simulink model "sl_subsys_sw1"  (Simulink 6.0)
settings: Solver=FixedStepDiscrete  SolverMode=SingleTasking  StartTime=0.0  StopTime=500  FixedStep=0.001  RelTol=1e-3
settings Model: CovMetricSettings=d  Creator=The MathWorks Inc.  LastModifiedBy=batserve  ExtModeAutoUpdateStatusClock=off
settings DataIOCC: SignalLoggingName=sigsOut
settings OptimizationCC: BlockReduction=off  BooleanDataType=off
settings DebuggingCC: CheckExecutionContextPreStartOutputMsg=on  CheckExecutionContextRuntimeOutputMsg=on  SolverPrmCheckMsg=none
settings HardwareCC: TargetUnknown=on

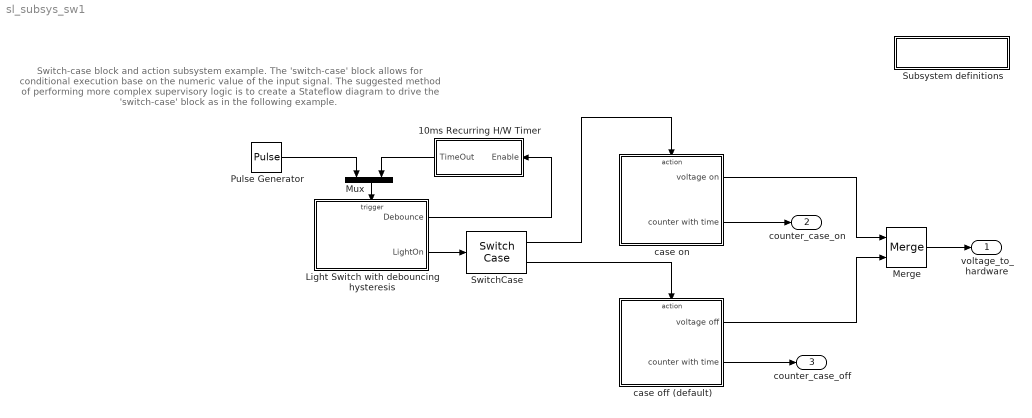
== system sl_subsys_sw1 ==
  note: Switch-case block and action subsystem example.
      |
      | The 'switch-case' block allows for conditional execution base on the numeric value
      | of the input signal. The suggested method of performing more complex supervisory
      | logic is to create a Stateflow diagram to drive the 'switch-case' block as in the
      | following example.
  " Subsystem definitions" : Subsystem  PropExecContextAcrossSSBoundary=on
      settings: OpenFcn=helpview([matlabroot,'/toolbox/simulink/simdemos/sl_subsys_definitions.html']);
      mask Display: disp('Subsystem\ndefinitions')
  10ms Recurring H/W Timer : Subsystem  Orientation=left  PropExecContextAcrossSSBoundary=on
  Light Switch with debouncing hysteresis : Stateflow chart  TreatAsAtomicUnit=on  PropExecContextAcrossSSBoundary=on
  Merge : Merge
  Mux : Mux  Orientation=down  Inputs=2
  Pulse Generator : DiscretePulseGenerator  Period=[64]  PulseWidth=[1]  PhaseDelay=1
  SwitchCase : SwitchCase
  case off (default) : Subsystem  TreatAsAtomicUnit=on  PropExecContextAcrossSSBoundary=on
  case on : Subsystem  TreatAsAtomicUnit=on  PropExecContextAcrossSSBoundary=on
  voltage_to_hardware : Outport
  counter_case_on : Outport  Port=2
  counter_case_off : Outport  Port=3
  wires:
  SwitchCase/1 -> case on/Action
  case on/1(voltage on) -> Merge/1
  case off (default)/1(voltage off) -> Merge/2
  Merge/1 -> voltage_to_hardware/1
  case on/2(counter with time) -> counter_case_on/1
  case off (default)/2(counter with time) -> counter_case_off/1
  Light Switch with debouncing hysteresis/2(LightOn) -> SwitchCase/1
  Light Switch with debouncing hysteresis/1(Debounce) -> 10ms Recurring H/W Timer/1(Enable)
  Mux/1 -> Light Switch with debouncing hysteresis/Trigger
  Pulse Generator/1 -> Mux/1
  10ms Recurring H/W Timer/1(TimeOut) -> Mux/2
  SwitchCase/2 -> case off (default)/Action

== system sl_subsys_sw1/ Subsystem definitions ==

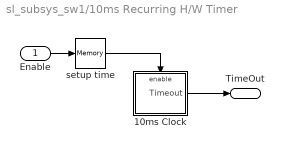
== system sl_subsys_sw1/10ms Recurring H/W Timer ==
  Enable : Inport  Port=1  LatchInput=off
  10ms Clock : Subsystem  TreatAsAtomicUnit=on  PropExecContextAcrossSSBoundary=on
  setup time : Memory  InheritSampleTime=on
  TimeOut : Outport
  wires:
  Enable/1 -> setup time/1
  10ms Clock/1(Timeout) -> TimeOut/1
  setup time/1 -> 10ms Clock/Enable

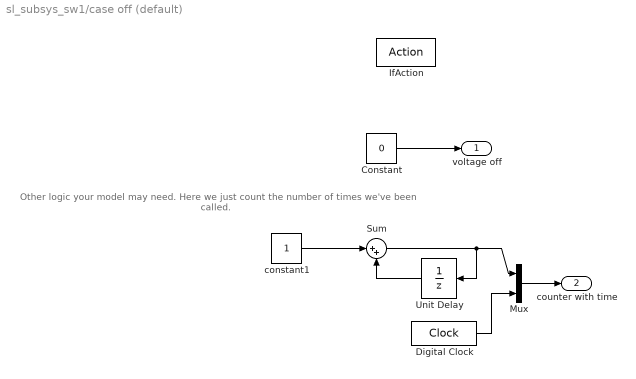
== system sl_subsys_sw1/case off (default) ==
  note: Other logic your model may need. Here we just count the number
      | of times we've been called.
  IfAction : ActionPort  ActionType=default
  Constant : Constant  Value=0
  Digital Clock : DigitalClock
  Mux : Mux  Inputs=2
  Sum : Sum  Inputs=|++  SaturateOnIntegerOverflow=on  InputSameDT=on
  Unit Delay : UnitDelay  Orientation=left
  constant1 : Constant
  voltage off : Outport
  counter with time : Outport  Port=2
  wires:
  Digital Clock/1 -> Mux/2
  Mux/1 -> counter with time/1
  Unit Delay/1 -> Sum/2
  constant1/1 -> Sum/1
  Sum/1 -> Unit Delay/1, Mux/1
  Constant/1 -> voltage off/1

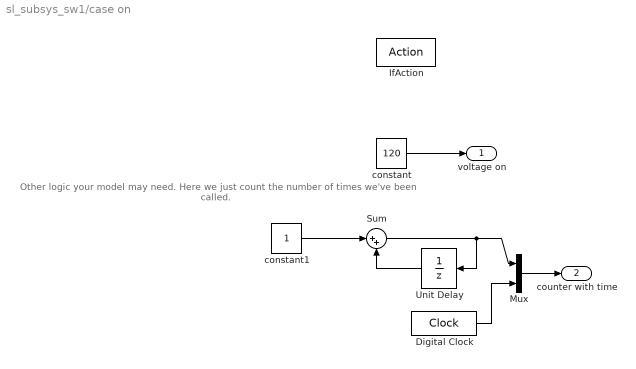
== system sl_subsys_sw1/case on ==
  note: Other logic your model may need. Here we just count the number
      | of times we've been called.
  IfAction : ActionPort  ActionType=case
  Digital Clock : DigitalClock
  Mux : Mux  Inputs=2
  Sum : Sum  Inputs=|++  SaturateOnIntegerOverflow=on  InputSameDT=on
  Unit Delay : UnitDelay  Orientation=left
  constant : Constant  Value=120
  constant1 : Constant
  voltage on : Outport
  counter with time : Outport  Port=2
  wires:
  Digital Clock/1 -> Mux/2
  Mux/1 -> counter with time/1
  Unit Delay/1 -> Sum/2
  constant1/1 -> Sum/1
  Sum/1 -> Mux/1, Unit Delay/1
  constant/1 -> voltage on/1

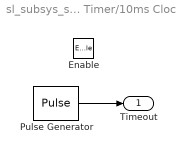
== system sl_subsys_sw1/10ms Recurring H/W Timer/10ms Clock ==
  Enable : EnablePort  StatesWhenEnabling=reset
  Pulse Generator : DiscretePulseGenerator  Amplitude=-1  Period=10  PulseWidth=5
  Timeout : Outport  OutputWhenDisabled=reset  InitialOutput=0
  wires:
  Pulse Generator/1 -> Timeout/1

== stateflow chart Light Switch with debouncing hysteresis ==
  settings: executeAtInitialization=1
  state On
    LightOn = 1;
  state Off
    LightOn = 0;
  state Debounce
    state Off
    state On
  On -> Debounce.Off : toggle
  Off -> Debounce.On : toggle
  (default) -> Off
  Debounce.On -> Off : toggle
  Debounce.On -> On : after(5,TimeOut)
  Debounce.Off -> On : toggle
  Debounce.Off -> Off : after(3,TimeOut)
  data: Debounce output State; LightOn output boolean
  events: toggle input RISING_EDGE_EVENT; TimeOut input RISING_EDGE_EVENT
